simulink model "SimulinkModel"  (R2025b)
settings: Solver=VariableStepAuto  StartTime=0.0  StopTime=360  FixedStep=0.10  MaxStep=5  MinStep=0.1  RelTol=0.5e-5  AbsTol=1e-5
values from neighbouring files (symbols this model uses):
  clock_drift_rate = 0.5    [run_simulink.m]
  w_earth = [0; 0; 7.2921159 * 10^(-5)]    [run_simulink.m]
undefined symbols (not defined in the file or in its folder): accelCorrectionInterval, baroCorrectionInterval, deg, gpsCorrectionInterval, IAU, IMUPropInterval, magCorrectionInterval, R_vec, rad, s, WMM2025
libraries: aerolibtransform2 x7, matrix_library x3, aerolibconvert2 x2, aerolibutil x2, aerolibsatdyn x1, aerolibnav x1, aerolibgravity2 x1, vrlib x1
(part 2 of 2)

== matlab function SimulinkModel/Embedded Computer/Enabled Subsystem/Example Q-Mekf/GPS Update/MATLAB Function ==
  data: oldState input; oldP input; state output; gps_sens input; R_vec input; P output; oldlastCalcTimes input; gps_correction_interval input; clock input; lastCalcTimes output
function [state, P, lastCalcTimes] = fcn(oldState, oldP, gps_sens, R_vec, oldlastCalcTimes, gps_correction_interval, clock)

lastCalcTimes = oldlastCalcTimes;

if clock - lastCalcTimes(4) >= gps_correction_interval

    H_gps = [zeros(3), zeros(3), eye(3), zeros(3), zeros(3), zeros(3), zeros(3, 1)];
    
    h_gps = oldState(8:10);
    
    R = diag(R_vec(7:9));
    
    [state, P] = residualErrorInject(oldState, oldP, gps_sens, H_gps, h_gps, R);
else
    state = oldState;
    P = oldP;
end
